simulink library "Storage_Type_11"  (R2018b)
settings: Solver=ode45  StartTime=0.0  StopTime=10.0  RelTol=1e-3  EnableMultiTasking=on
undefined symbols (not defined in the file): heater1end, heater1start, path_carnot
libraries: carnot x8
settings Model: Creator=bernd.hafner  LastModifiedBy=drhf
settings DataIOCC: LimitDataPoints=on  SaveFormat=Array  SignalLoggingSaveFormat=ModelDataLogs
settings OptimizationCC: ExpressionDepthLimit=2147483647  LifeSpan=inf
settings DebuggingCC: UnderspecifiedInitializationDetection=Classic  MergeDetectMultiDrivingBlocksExec=none  SolverPrmCheckMsg=warning  FcnCallInpInsideContextMsg=warning  StateNameClashWarn=warning  SFUnexpectedBacktrackingDiag=warning  SFNoUnconditionalDefaultTransitionDiag=warning  SFExecutionAtInitializationDiag=none
settings HardwareCC: ProdBitPerPointer=32  ProdBitPerSizeT=32  ProdBitPerPtrDiffT=32  ProdLargestAtomicFloat=None  ProdIntDivRoundTo=Undefined  ProdEndianess=Unspecified  ProdWordSize=32  ProdHWDeviceType=32-bit Generic
settings ModelReferenceCC: PropagateSignalLabelsOutOfModel=off
settings SFSimCC: SimUseLocalCustomCode=off
settings RTWCC: RTWUseLocalCustomCode=off
settings CodeAppCC: StateflowObjectComments=on
settings GRTTargetCC: TargetLangStandard=C89/C90 (ANSI)  GeneratePreprocessorConditionals=Disable all  CombineOutputUpdateFcns=off  GRTInterface=on
settings ConfigComp: CovMetricSettings=dw  CovHtmlReporting=on  CovSaveCumulativeToWorkspaceVar=on  CovSaveSingleToWorkspaceVar=on  CovExternalEMLEnable=off

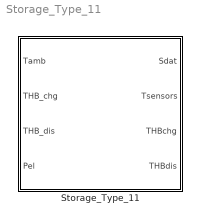
== system Storage_Type_11 ==
  Storage_Type_11 : Subsystem  mask(Buffer storage tank){t0=10, hgt=1.7684, stgtype=11, tini=[10 10 10 10 10 10 10 10 10 10], mpts=[1 2 3 4 5 6 7 8 9 10], PathName=fullfile(path_carnot('libsl'), 'Storage', 'Thermal', 'Storage_Type_11', 'parameter_set'), FileName='StorageType11_500_L.mat', userPath=off, userParam=off, uwall=1, ubot=1, utop=1, axcond=1, volume=0.5, dia=0.6, standing=standing cylinder, nodes=10, mpoints=10, Tsensor=0.5, vTpiece=0.004, pipe1inlet=1, pipe1outlet=0, pipe1dia=0.03, pipe2inlet=0.1, pipe2outlet=1, pipe2dia=0.03, heater1start=heater1start, heater1end=heater1end}
      mask prompts: t0 "Initial temperature (vector or scalar) in °C"; hgt "Height of storage in m"; stgtype "Storage Type"; tini "Start temperatures of nodes in °C"; mpts "Index to measured nodes"; PathName "Path"; FileName "Parameter set"; userPath "Edit path and name of parameter set"; userParam "User defined parameters"; uwall "Heat transfer coefficient to ambient [W/m²K]"; ubot "Heat transfer coefficient to ambient bottom [W/m²K]"; utop "Heat transfer coefficient to ambient top [W/m²K]"; axcond "Effective thermal conductivity [W/m/K]"; volume "Volume [m³]"; dia "Diameter [m]"; standing "Position"; nodes "Number of nodes"; mpoints "Number of node temperatures (for display)"; Tsensor "Temperature sensor position (0..1, 0 = bottom, 1 = top)"; vTpiece "Volume of the flowline with T-piece [m³]"; pipe1inlet "relative height of inlet, range from 0 (= bottom) to 1 (= top)"; pipe1outlet "relative height of outlet, range from 0 (= bottom) to 1 (= top)"; pipe1dia "Diameter of pipe in m"; pipe2inlet "relative height of inlet, range from 0 (= bottom) to 1 (= top)"; pipe2outlet "relative height of outlet, range from 0 (= bottom) to 1 (= top)"; pipe2dia "Diameter of pipe in m"; heater1start "relative height start heating zone"; heater1end "relative height end heating zone"
      mask help:
      | Buffer storage for heating circuits. The buffer ist connected at "3 points".
      | The flowline of the heat generators (charing port) is connected with the flowline of the load (discharging port) and the buffer via a T-piece.
      | The return of the load and the heat generators is connected to the lower part of the storage.
      mask init:
      | [ok, param] = CarnotCallbacks_StorageConf('SetParam',stgtype,gcbh,PathName,FileName);
      | 
      | set_param([gcb,'/Pipe with T-piece'],'volume',num2str(vTpiece))
      mask Help: web(fullfile(path_carnot('help'),'Storage_Type_11.html'),'-helpbrowser')
      mask TypeOptions hgt: Pipe_Connection_1/hgt | Pipe_Connection_2/hgt
      mask TypeOptions stgtype: CreateSdat/stgtype
      mask TypeOptions tini: sfun_storageTnodes/tini
      mask TypeOptions mpts: select_T/Indices
      mask Callback userPath: [ok, param] = CarnotCallbacks_StorageConf('UserEdit',1,gcbh);
      mask Callback userParam: [ok, param] = CarnotCallbacks_StorageConf('UserEdit',1,gcbh);
      mask TypeOptions uwall: sfun_storageTnodes/uloss
      mask TypeOptions ubot: sfun_storageTnodes/ubot
      mask TypeOptions utop: sfun_storageTnodes/utop
      mask TypeOptions axcond: sfun_storageTnodes/cond
      mask TypeOptions volume: sfun_storageTnodes/volume | CreateSdat/volume
      mask TypeOptions dia: sfun_storageTnodes/dia | Pipe_Connection_1/dstg | Pipe_Connection_2/dstg
      mask TypeOptions standing: sfun_storageTnodes/standing
      mask TypeOptions nodes: sfun_storageTnodes/nodes | select_T/InputPortWidth | HX_EN12977_1/nodes | HX_EN12977_2/nodes | HX_EN12977_3/nodes | Pipe_Connection_1/nodes | Pipe_Connection_2/nodes | Pipe_Connection_3/nodes
      mask TypeOptions Tsensor: T_Sensor_Surface/pos
      mask TypeOptions pipe1inlet: Pipe_Connection_1/h_in
      mask TypeOptions pipe1outlet: Pipe_Connection_1/h_out
      mask TypeOptions pipe1dia: Pipe_Connection_1/dpipe
      mask TypeOptions pipe2inlet: Pipe_Connection_2/h_in
      mask TypeOptions pipe2outlet: Pipe_Connection_2/h_out
      mask TypeOptions pipe2dia: Pipe_Connection_2/dpipe
      mask TypeOptions heater1start: Electric_Heating_1/hin
      mask TypeOptions heater1end: Electric_Heating_1/hout
      mask DialogControl Container14 Prompt: Infos
      mask DialogControl ParameterGroupVar Prompt: Picking a parameter set
      mask DialogControl Control3 Prompt: Carnot public data
      mask DialogControl Control3 Callback: [ok, file] = CarnotCallbacks_StorageConf('GetFilename',1,gcbh,'public');
      mask DialogControl Control4 Prompt: Carnot internal data
      mask DialogControl Control4 Callback: [ok, file] = CarnotCallbacks_StorageConf('GetFilename',1,gcbh,'internal');
      mask DialogControl Control2 Prompt: Selected path
      mask DialogControl Control2 Callback: [ok, file] = CarnotCallbacks_StorageConf('GetFilename',1,gcbh,'selected');
      mask DialogControl Container4 Prompt: Parameter values
      mask DialogControl Container6 Prompt: Storage
      mask DialogControl Container8 Prompt: Connections
      mask DialogControl Container9 Prompt: Charging pipe
      mask DialogControl Container12 Prompt: Discharging pipe
      mask DialogControl Container13 Prompt: Electric Heating
      mask DialogControl Container15 Prompt: Heater 1
      mask DialogControl Control6 Prompt: Save in Carnot internal data
      mask DialogControl Control6 Callback: [ok, param] = CarnotCallbacks_StorageConf('SaveFilename',1,gcbh,'internal','STG');
      mask DialogControl Control5 Prompt: Save in selected path
      mask DialogControl Control5 Callback: [ok, param] = CarnotCallbacks_StorageConf('SaveFilename',1,gcbh,'selected','STG');
      mask Display:
      | % user defined picture file
      | namestr = 'BufferStorage3pt';
      | picfile = fullfile(path_carnot('intlibsl'), 'Storage','Thermal', ...
      |     namestr,'parameter_set', [namestr, '.jpg']);
      | 
      | % show internal picture if defined
      | pic = false;
      | if  ~BlockIsInCarnotLibrary       % if not located in library
      |     if exist(picfile, 'file')
      |         image(imread(picfile), [0.25, 0, 0.45, 1])
      |         set_param(gcb, 'BackgroundColor', 'White')
      |         pic = true;
      |     end
      | end
      | 
      | % show public picture
      | if ~pic
      |     set_param(gcb, 'BackgroundColor', 'Red')
      |     plot([40,30,30,40,60,70,70,60,40]/120+0.1,[90,80,10,0,0,10,80,90,90]/110+0.05, ...
      |         [80,20]/120+0.1,[100,100]/110+0.05, ...
      |         [50,50]/120+0.1,[90,100]/110+0.05, ...
      |         [30,20]/120+0.1,[13,13]/110+0.05, ...
      |         [80,70]/120+0.1,[13,13]/110+0.05,...
      |         [30,50,50,30]/120+0.1,[62,62,60,60]/110,...
      |         [30,27,27,30]/120+0.1,[64,64,58,58]/110)
      | end

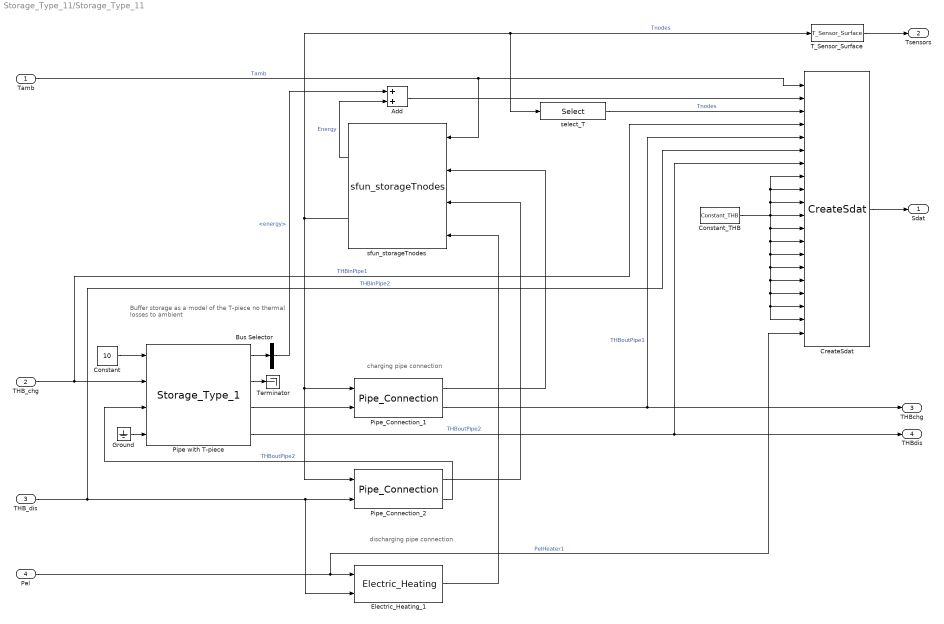
== system Storage_Type_11/Storage_Type_11 ==
  note: discharging pipe connection
  note: charging pipe connection
  note: Buffer storage as a model of the T-piece
      | no thermal losses to ambient
  Tamb : Inport
  THB_chg : Inport  Port=2
  THB_dis : Inport  Port=3
  Pel : Inport  Port=4
  Add : Sum
  Bus Selector : BusSelector  OutputSignals=energy
  Constant : Constant  Value=10
  Constant_THB : carnot/Source/Simple/Constant_THB  t=20  mdot=0  p=1e5  mID=No Pressure Drop  fluid=Water  mix=0  mix2=0  mix3=0  dia=0.02  hgt=0
      settings: SourceProductName=Carnot
  CreateSdat : carnot/Basic/Thermal_Models/CreateSdat  volume=volume  stgtype=stgtype
      settings: SourceProductName=Carnot
  Electric_Heating_1 : carnot/Storage/Thermal/Storage_Ports/Electric_Heating  hin=heater1start  hout=heater1end  nodes=nodes
      settings: SourceProductName=Carnot
  Ground : Ground
  Pipe with T-piece : carnot/Storage/Thermal/Storage_Type_1  t0=10  hgt=0.5093  stgtype=1  tini=10  mpts=1  PathName=fullfile(path_carnot('libsl'),'Storage','Thermal','Storage_Type_11','parameter_set')  FileName='<user defined>'  userPath=off  userParam=on  uwall=0  ubot=0  utop=0  axcond=0  volume=0.004  dia=0.1  standing=standing cylinder  nodes=1  mpoints=1  Tsensor=0.5  pipe1inlet=1  pipe1outlet=0  pipe1dia=0.03  pipe2inlet=0  pipe2outlet=1  pipe2dia=0.03  heater1start=0.6  heater1end=0.65
      settings: SourceProductName=Carnot
  Pipe_Connection_1 : carnot/Storage/Thermal/Storage_Ports/Pipe_Connection  h_in=pipe1inlet  h_out=pipe1outlet  hgt=hgt  dpipe=pipe1dia  dstg=dia  height=-1.7684  nodes=nodes
      settings: SourceProductName=Carnot
  Pipe_Connection_2 : carnot/Storage/Thermal/Storage_Ports/Pipe_Connection  h_in=pipe2inlet  h_out=pipe2outlet  hgt=hgt  dpipe=pipe2dia  dstg=dia  height=1.5916  nodes=nodes
      settings: SourceProductName=Carnot
  T_Sensor_Surface : carnot/Control/T_Sensor_Surface  pos=Tsensor  tdel=10  t0=mean(tini)
      settings: SourceProductName=Carnot
  Terminator : Terminator
  select_T : Selector  InputPortWidth=nodes  IndexOptions=Index vector (dialog)  Indices=[1 2 3 4 5 6 7 8 9 10]  OutputSizes=1
  sfun_storageTnodes : carnot/Basic/Thermal_Models/sfun_storageTnodes  uloss=uwall  ubot=ubot  utop=utop  cond=axcond  volume=volume  dia=dia  standing=standing cylinder  tini=tini  nodes=nodes  nconnect=3  elimthermocline=2  condinvtc=1e5
      settings: SourceProductName=Carnot
  Sdat : Outport
  Tsensors : Outport  Port=2
  THBchg : Outport  Port=3
  THBdis : Outport  Port=4
  wires:
  Pipe with T-piece/3 -> Pipe_Connection_1/2
  Pipe with T-piece/1 -> Bus Selector/1
  Pipe with T-piece/2 -> Terminator/1
  Constant/1 -> Pipe with T-piece/1
  Constant_THB/1 -> CreateSdat/8, CreateSdat/9, CreateSdat/10, CreateSdat/11, CreateSdat/12, CreateSdat/13, CreateSdat/14, CreateSdat/15, CreateSdat/19, CreateSdat/18, CreateSdat/17, CreateSdat/16
  T_Sensor_Surface/1 -> Tsensors/1
  Pipe_Connection_1/1 -> sfun_storageTnodes/2
  CreateSdat/1 -> Sdat/1
  sfun_storageTnodes/2 -> Pipe_Connection_2/1, Pipe_Connection_1/1, T_Sensor_Surface/1, select_T/1  "Tnodes"
  select_T/1 -> CreateSdat/3  "Tnodes"
  Tamb/1 -> CreateSdat/1, sfun_storageTnodes/1  "Tamb"
  Pipe_Connection_2/1 -> sfun_storageTnodes/3
  sfun_storageTnodes/1 -> Add/2  "Energy"
  THB_chg/1 -> Pipe with T-piece/2, CreateSdat/4  "THBinPipe1"
  Pipe with T-piece/4 -> CreateSdat/7, THBdis/1  "THBoutPipe2"
  Pipe_Connection_1/2 -> THBchg/1, CreateSdat/5  "THBoutPipe1"
  Pipe_Connection_2/2 -> Pipe with T-piece/3  "THBoutPipe2"
  Add/1 -> CreateSdat/2
  Bus Selector/1 -> Add/1  "<energy>"
  Pel/1 -> Electric_Heating_1/1, CreateSdat/20  "PelHeater1"
  THB_dis/1 -> Electric_Heating_1/2, Pipe_Connection_2/2, CreateSdat/6  "THBinPipe2"
  Electric_Heating_1/1 -> sfun_storageTnodes/4
  Ground/1 -> Pipe with T-piece/4
